simulink library "csu_arg_aimpoint_roll_guidance_lib"  (R2014b)
settings: Solver=ode45  StartTime=0.0  StopTime=10.0  RelTol=1e-3
values from neighbouring files (symbols this model uses):
  arg_aimpoint_body_vector = [0 0 1]    [csu_arg_aimpoint_roll_guidance_init.m]
  arg_roll_body_pointing_vector = [-cosd(60) -sind(60) 0]    [csu_arg_aimpoint_roll_guidance_init.m]
  arg_roll_inertial_target_vector = [0.9774   -0.2057   -0.0482]    [csu_arg_aimpoint_roll_guidance_init.m]
libraries: util_common_lib x15, simulink x6, util_quat_lib x2, util_extra_lib x2, util_info_lib x1
settings Model: Creator=ianmga  LastModifiedBy=mstewart

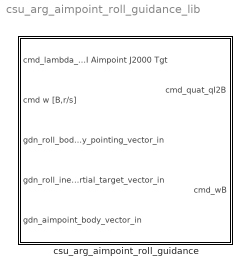
== system csu_arg_aimpoint_roll_guidance_lib ==
  csu_arg_aimpoint_roll_guidance : Subsystem

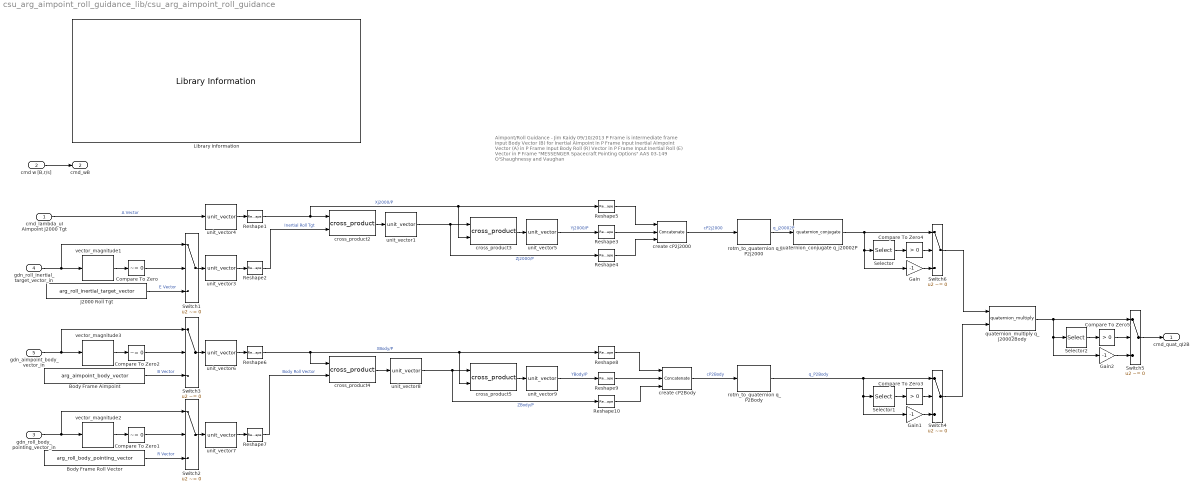
== system csu_arg_aimpoint_roll_guidance_lib/csu_arg_aimpoint_roll_guidance ==
  note: Aimpont/Roll Guidance - Jim Kaidy 09/10/2013
      | P Frame is intermediate frame
      | Input Body Vector (B) for Inertial Aimpoint in P Frame
      | Input Inertial Aimpoint Vector (A) in P Frame
      | Input Body Roll (R) Vector in P Frame
      | Input Inertial Roll (E) Vector in P Frame
      | "MESSENGER Spacecraft Pointing Options" AAS 03-149
      | O'Shaughnessy and Vaughan
  cmd_lambda_uI Aimpoint J2000 Tgt : Inport
  cmd w [B,r/s] : Inport  Port=2
  gdn_roll_body_pointing_vector_in : Inport  Port=3
  gdn_roll_inertial_target_vector_in : Inport  Port=4
  gdn_aimpoint_body_vector_in : Inport  Port=5
  "Body Frame Aimpoint " : Constant  Value=arg_aimpoint_body_vector
  Body Frame Roll Vector : Constant  Value=arg_roll_body_pointing_vector
  Compare To Zero : simulink/Logic and Bit Operations/Compare To Zero  relop=~=  OutDataTypeStr=boolean
  Compare To Zero1 : simulink/Logic and Bit Operations/Compare To Zero  relop=~=  OutDataTypeStr=boolean
  Compare To Zero2 : simulink/Logic and Bit Operations/Compare To Zero  relop=~=  OutDataTypeStr=boolean
  Compare To Zero3 : simulink/Logic and Bit Operations/Compare To Zero  relop=>  OutDataTypeStr=boolean
  Compare To Zero4 : simulink/Logic and Bit Operations/Compare To Zero  relop=>  OutDataTypeStr=boolean
  Compare To Zero5 : simulink/Logic and Bit Operations/Compare To Zero  relop=>  OutDataTypeStr=boolean
  Gain : Gain  Gain=-1
  Gain1 : Gain  Gain=-1
  Gain2 : Gain  Gain=-1
  J2000 Roll Tgt : Constant  Value=arg_roll_inertial_target_vector
  Library Information : util_info_lib/Library Information  owner='NONE'
  Reshape{1..10} (10 alike) : Reshape  OutputDimensionality=Column vector (2-D)
  Selector : Selector  InputPortWidth=4  Indices=[4]
  Selector1 : Selector  InputPortWidth=4  Indices=[4]
  Selector2 : Selector  InputPortWidth=4  Indices=[4]
  Switch1 : Switch  Criteria=u2 ~= 0  Threshold=0.5
  Switch2 : Switch  Criteria=u2 ~= 0  Threshold=0.5
  Switch3 : Switch  Criteria=u2 ~= 0  Threshold=0.5
  Switch4 : Switch  Criteria=u2 ~= 0
  Switch5 : Switch  Criteria=u2 ~= 0
  Switch6 : Switch  Criteria=u2 ~= 0
  create cP2Body : Concatenate  NumInputs=3  Mode=Multidimensional array  ConcatenateDimension=2
  create cP2j2000 : Concatenate  NumInputs=3  Mode=Multidimensional array  ConcatenateDimension=2
  cross_product{2..5} (4 alike) : util_common_lib/cross_product  SystemSampleTime=-1
  quaternion_conjugate q_j20002P : util_quat_lib/quaternion_conjugate  SystemSampleTime=-1
  quaternion_multiply q_j20002Body : util_quat_lib/quaternion_multiply  SystemSampleTime=-1
  rotm_to_quaternion q_P2Body : util_extra_lib/rotm_to_quaternion
  rotm_to_quaternion q_P2j2000 : util_extra_lib/rotm_to_quaternion
  unit_vector{1,3..9} (8 alike) : util_common_lib/unit_vector  SystemSampleTime=-1
  vector_magnitude1 : util_common_lib/vector_magnitude  SystemSampleTime=-1
  vector_magnitude2 : util_common_lib/vector_magnitude  SystemSampleTime=-1
  vector_magnitude3 : util_common_lib/vector_magnitude  SystemSampleTime=-1
  cmd_quat_qI2B : Outport
  cmd_wB : Outport  Port=2
  wires:
  Switch4/1 -> quaternion_multiply q_j20002Body/2
  rotm_to_quaternion q_P2Body/1 -> Switch4/1, Selector1/1, Gain1/1  "q_P2Body"
  Gain1/1 -> Switch4/3
  Selector1/1 -> Compare To Zero3/1
  Switch6/1 -> quaternion_multiply q_j20002Body/1
  Gain/1 -> Switch6/3
  cmd w [B,r/s]/1 -> cmd_wB/1
  create cP2j2000/1 -> rotm_to_quaternion q_P2j2000/1  "cP2j2000"
  Reshape5/1 -> create cP2j2000/1
  Reshape3/1 -> create cP2j2000/2
  Reshape4/1 -> create cP2j2000/3
  cross_product3/1 -> unit_vector5/1
  unit_vector1/1 -> Reshape4/1, cross_product3/1  "Zj2000/P"
  cross_product2/1 -> unit_vector1/1
  cmd_lambda_uI Aimpoint J2000 Tgt/1 -> unit_vector4/1  "A Vector"
  Reshape1/1 -> Reshape5/1, cross_product3/2, cross_product2/1  "Xj2000/P"
  unit_vector4/1 -> Reshape1/1
  unit_vector5/1 -> Reshape3/1  "Yj2000/P"
  unit_vector6/1 -> Reshape6/1
  gdn_roll_body_pointing_vector_in/1 -> vector_magnitude2/1, Switch2/1
  vector_magnitude2/1 -> Compare To Zero1/1
  Body Frame Roll Vector/1 -> Switch2/3  "R Vector"
  Switch2/1 -> unit_vector7/1
  Compare To Zero1/1 -> Switch2/2
  J2000 Roll Tgt/1 -> Switch1/3  "E Vector"
  gdn_roll_inertial_target_vector_in/1 -> Switch1/1, vector_magnitude1/1
  vector_magnitude1/1 -> Compare To Zero/1
  Compare To Zero/1 -> Switch1/2
  unit_vector3/1 -> Reshape2/1
  Reshape2/1 -> cross_product2/2  "Inertial Roll Tgt"
  Switch1/1 -> unit_vector3/1
  unit_vector7/1 -> Reshape7/1
  Reshape7/1 -> cross_product4/2  "Body Roll Vector"
  cross_product4/1 -> unit_vector8/1
  create cP2Body/1 -> rotm_to_quaternion q_P2Body/1  "cP2Body"
  Reshape8/1 -> create cP2Body/1
  Reshape9/1 -> create cP2Body/2
  Reshape10/1 -> create cP2Body/3
  cross_product5/1 -> unit_vector9/1
  unit_vector8/1 -> Reshape10/1, cross_product5/1  "ZBody/P"
  Reshape6/1 -> cross_product4/1, Reshape8/1, cross_product5/2  "XBody/P"
  unit_vector9/1 -> Reshape9/1  "YBody/P"
  rotm_to_quaternion q_P2j2000/1 -> quaternion_conjugate q_j20002P/1  "q_j20002P"
  quaternion_conjugate q_j20002P/1 -> Switch6/1, Gain/1, Selector/1
  Selector/1 -> Compare To Zero4/1
  gdn_aimpoint_body_vector_in/1 -> Switch3/1, vector_magnitude3/1
  vector_magnitude3/1 -> Compare To Zero2/1
  Switch3/1 -> unit_vector6/1
  Compare To Zero2/1 -> Switch3/2
  "Body Frame Aimpoint "/1 -> Switch3/3  "B Vector"
  Gain2/1 -> Switch5/3
  quaternion_multiply q_j20002Body/1 -> Selector2/1, Gain2/1, Switch5/1
  Selector2/1 -> Compare To Zero5/1
  Switch5/1 -> cmd_quat_qI2B/1
  Compare To Zero3/1 -> Switch4/2
  Compare To Zero4/1 -> Switch6/2
  Compare To Zero5/1 -> Switch5/2
